simulink library "Input_Silicon_Oil"  (Simulink 8.2)
settings: Solver=ode45  StartTime=0.0  StopTime=10.0  RelTol=1e-3
settings Model: Creator=lena.frank  LastModifiedBy=drhf

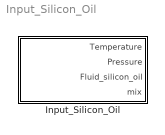
== system Input_Silicon_Oil ==
  Input_Silicon_Oil : Subsystem  mask(Input_Silicon_Oil){T=20, p=1e5}
      mask prompts: T "temperature (scalar or vector) [°C]"; p "pressure [Pa]"
      mask help: Input block for the material "Silicon_Oil". The relevant inputs for the calculation of the block can be specified as parameter in the mask
      mask Help: web(fullfile(path_carnot('help'),'input_material.html'),'-helpbrowser')

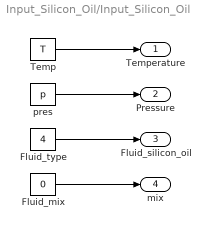
== system Input_Silicon_Oil/Input_Silicon_Oil ==
  Fluid_mix : Constant  Value=0
  Fluid_type : Constant  Value=4
  Temp : Constant  Value=T
  pres : Constant  Value=p
  Temperature : Outport
  Pressure : Outport  Port=2
  Fluid_silicon_oil : Outport  Port=3
  mix : Outport  Port=4
  wires:
  pres/1 -> Pressure/1
  Temp/1 -> Temperature/1
  Fluid_type/1 -> Fluid_silicon_oil/1
  Fluid_mix/1 -> mix/1
